simulink model "ROSmsg2PrescanPos"  (R2022b)
settings: Solver=VariableStepAuto  StartTime=0.0  StopTime=10.0  RelTol=1e-3
libraries: MainLibrary x3
settings Model: Creator=20211327  LastModifiedBy=20211327

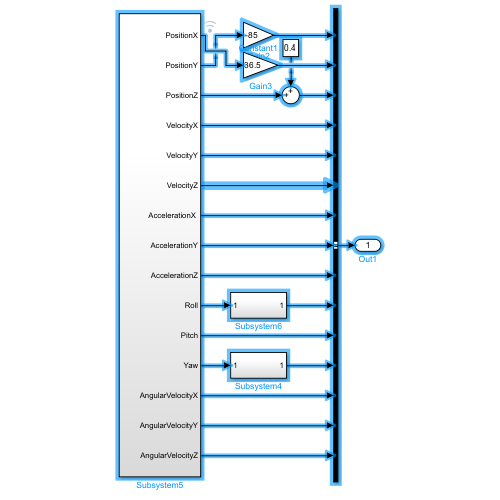
[thumbnail: Simulink's stored preview of the top-level diagram]
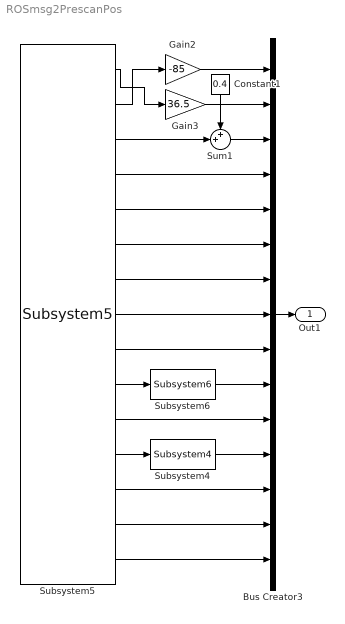
== system ROSmsg2PrescanPos ==
  Bus Creator3 : BusCreator  Inputs=15
  Constant1 : Constant  Value=0.4
  Gain2 : Gain  Gain=-85
  Gain3 : Gain  Gain=36.5
  Subsystem4 : MainLibrary/ROSmsg2PrescanPos/ROS msg to Prescan Pos/Subsystem4  SystemSampleTime=-1  VariantActivationTime=update diagram  Latency=0  AutoFrameSizeCalculation=off
      settings: SourceProductName=Custom_Prescan-ROS_Library
  Subsystem5 : MainLibrary/ROSmsg2PrescanPos/ROS msg to Prescan Pos/Subsystem5  SystemSampleTime=-1  VariantActivationTime=update diagram  Latency=0  AutoFrameSizeCalculation=off
      settings: SourceProductName=Custom_Prescan-ROS_Library
  Subsystem6 : MainLibrary/ROSmsg2PrescanPos/ROS msg to Prescan Pos/Subsystem6  SystemSampleTime=-1  VariantActivationTime=update diagram  Latency=0  AutoFrameSizeCalculation=off
      settings: SourceProductName=Custom_Prescan-ROS_Library
  Sum1 : Sum  Inputs=++|
  Out1 : Outport
  wires:
  Gain3/1 -> Bus Creator3/2
  Sum1/1 -> Bus Creator3/3
  Gain2/1 -> Bus Creator3/1
  Subsystem5/13 -> Bus Creator3/13
  Subsystem5/11 -> Bus Creator3/11
  Subsystem5/15 -> Bus Creator3/15
  Subsystem5/1 -> Gain3/1
  Bus Creator3/1 -> Out1/1
  Subsystem4/1 -> Bus Creator3/12
  Subsystem5/14 -> Bus Creator3/14
  Subsystem5/12 -> Subsystem4/1
  Subsystem6/1 -> Bus Creator3/10
  Constant1/1 -> Sum1/1
  Subsystem5/7 -> Bus Creator3/7
  Subsystem5/9 -> Bus Creator3/9
  Subsystem5/8 -> Bus Creator3/8
  Subsystem5/5 -> Bus Creator3/5
  Subsystem5/10 -> Subsystem6/1
  Subsystem5/2 -> Gain2/1
  Subsystem5/3 -> Sum1/2
  Subsystem5/4 -> Bus Creator3/4
  Subsystem5/6 -> Bus Creator3/6
